simulink model "LR4_MostKran_0"  (R2015b)
settings: Solver=FixedStepAuto  StartTime=0.0  StopTime=100.0  FixedStep=dT  RelTol=1e-3
values from neighbouring files (symbols this model uses):
  A = [0, 1, 0, 0;  0, 0, a23, 0;  0, 0, 0, 1;  0, 0, a43, 0]    [LR_4_MostKran.m]
  B = [0; b2; 0; b4]    [LR_4_MostKran.m]
  C = [1, 0, 0, 0; 0, 1, 0, 0; 0, 0, 1, 0; 0, 0, 0, 1]    [LR_4_MostKran.m]
  D = [0; 0; 0; 0]    [LR_4_MostKran.m]
  X0 = [0; 0; 0; 0]    [LR_4_MostKran.m]
undefined symbols (not defined in the file or in its folder): sigbuilder_block
settings Model: Creator=Сергей  LastModifiedBy=Сергей

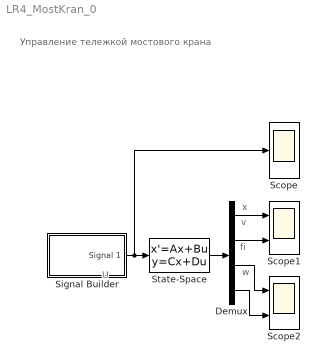
== system LR4_MostKran_0 ==
  note: w
  note: fi
  note: v
  note: x
  note: U
  note: Управление тележкой мостового крана
  Demux : Demux
  Scope : Scope
  Scope1 : Scope  NumInputPorts=2
  Scope2 : Scope  NumInputPorts=2
  Signal Builder : Subsystem  Tag=STV Subsys  LoadFcn=sigbuilder_block('load');  StartFcn=sigbuilder_block('start');  StopFcn=sigbuilder_block('stop');  ClipboardFcn=sigbuilder_block('clipboard');  mask(Sigbuilder block){}
      mask help: Simulink:masks:SigbuilderBlock_MD
      mask init:
      | if ~strcmp(get_param(bdroot(gcbh),'SimulationStatus'),'stopped') tuvar = sigbuilder_block('maskInit'); end
      settings: CopyFcn=sigbuilder_block('copy');  DeleteFcn=sigbuilder_block('delete');  ModelCloseFcn=sigbuilder_block('modelClose');  PreSaveFcn=sigbuilder_block('preSave');  PauseFcn=sigbuilder_block('pause');  ContinueFcn=sigbuilder_block('continue');  NameChangeFcn=sigbuilder_block('namechange');  OpenFcn=sigbuilder_block('open',[63.75 114.75 550.5 399.75 ]);  CloseFcn=sigbuilder_block('close');
      mask Display: plot(0, 0, 100, 100,[2, 2, 32, 32, 2], [68, 8, 8, 68, 68],[32, 2], [38, 38], [32, 19, 2],[53, 60, 44], [32, 17, 17, 2],[16, 16, 31, 31]);txt = getActiveGroup(gcbh);text(2, 100, txt,'verticalAlignment', 'top');
  State-Space : StateSpace  A=A  B=B  C=C  D=D  X0=X0
  wires:
  Signal Builder/1(Signal 1) -> Scope/1, State-Space/1
  State-Space/1 -> Demux/1
  Demux/1 -> Scope1/1
  Demux/2 -> Scope1/2
  Demux/3 -> Scope2/1
  Demux/4 -> Scope2/2

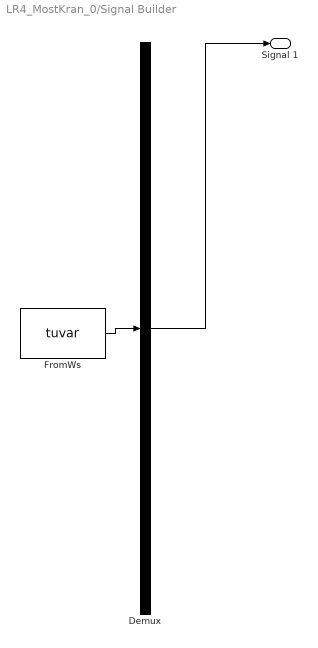
== system LR4_MostKran_0/Signal Builder ==
  Demux : Demux  Tag=STV Demux  Outputs=1
  FromWs : FromWorkspace  Tag=STV FromWs  VariableName=tuvar  SampleTime=0
      SigBuilderData=|
      | common.afterFinalStr = 'Extrapolate'
      | common.sampleTime = 0
      | dataSet.timeRange = [0 100]
      | dataSet.name = 'Group 1'
      | sbobj.Groups.Name = 'Group 1'
      | sbobj.Groups.Signals.Name = 'Signal 1'
      | sbobj.Groups.Signals.XData = [0 1 1 10 10 19 19 100]
      | sbobj.Groups.Signals.YData = [0 0 40 40 -40 -40 0 0]
      | sbobj.Groups.TimeRange = [0 100]
  Signal 1 : Outport  Tag=STV Outport
  wires:
  Demux/1 -> Signal 1/1
  FromWs/1 -> Demux/1
